simulink model "HINF"  (R2025b)
settings: Solver=VariableStepAuto  StartTime=0.0  StopTime=5.0  RelTol=1e-3
libraries: cstblocks x2
settings Model: Creator=salvo  LastModifiedBy=salvo

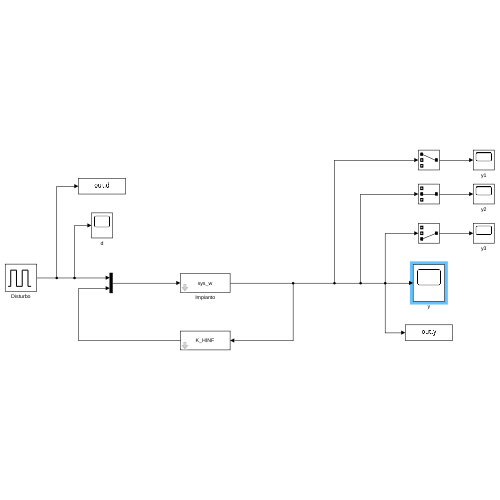
[thumbnail: Simulink's stored preview of the top-level diagram]
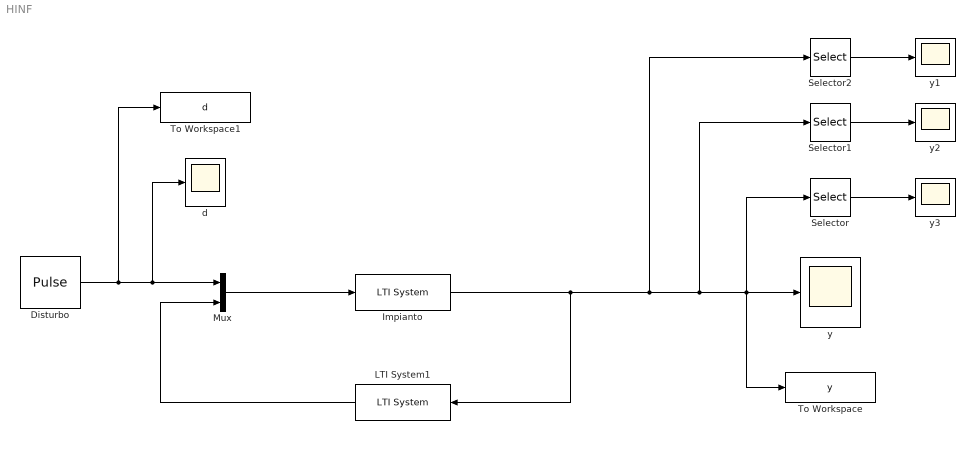
== system HINF ==
  Disturbo : DiscretePulseGenerator  PulseType=Time based  Amplitude=0.5  Period=30  PulseWidth=0.1
  Impianto : cstblocks/LTI System  sys=sys_w  IC=[]  PadeOrder=0
  LTI System1 : cstblocks/LTI System  sys=K_HINF  IC=[]  PadeOrder=0
  Mux : Mux  Inputs=2
  Selector : Selector  InputPortWidth=3  IndexOptions=Index vector (dialog)  Indices=[3]  OutputSizes=1
  Selector1 : Selector  InputPortWidth=3  IndexOptions=Index vector (dialog)  Indices=[2]  OutputSizes=1
  Selector2 : Selector  InputPortWidth=3  IndexOptions=Index vector (dialog)  Indices=[1]  OutputSizes=1
  To Workspace : ToWorkspace  VariableName=y  SaveFormat=Timeseries  SampleTime=-1
  To Workspace1 : ToWorkspace  VariableName=d  SaveFormat=Timeseries  SampleTime=-1
  d : Scope
      settings: ActiveDisplayYMinimum=0.282988154335187  ActiveDisplayYMaximum=0.68939084247621918
  y{,1..3} (4 alike) : Scope
      y settings: ActiveDisplayYMinimum=-0.15342076846596353  ActiveDisplayYMaximum=0.233629410715972
      y1 settings: ActiveDisplayYMinimum=-0.15646107331535819  ActiveDisplayYMaximum=0.06398331657512682  DataLoggingVariableName=ScopeData4
      y2 settings: ActiveDisplayYMinimum=-0.018254553713478706  ActiveDisplayYMaximum=0.036891595755091364  DataLoggingVariableName=ScopeData5
      y3 settings: ActiveDisplayYMinimum=0.25868528928511036  ActiveDisplayYMaximum=1.3909079750846918  DataLoggingVariableName=ScopeData3
  wires:
  Mux/1 -> Impianto/1
  LTI System1/1 -> Mux/2
  Impianto/1 -> LTI System1/1, Selector2/1, Selector1/1, To Workspace/1, Selector/1, y/1
  Selector2/1 -> y1/1
  Selector1/1 -> y2/1
  Selector/1 -> y3/1
  Disturbo/1 -> To Workspace1/1, d/1, Mux/1
